simulink model "VTOL_V4_Final_LANDING"  (R2022b)
settings: Solver=ode23s  StartTime=0.0  StopTime=20  RelTol=1e-3
values from neighbouring files (symbols this model uses):
  x0 = [Cruise.landingConditions.uvw.Data(end,1) ... (first row only)    [Plot_Transition.m]    (also in Start.m = [21.9999986140590)
undefined symbols (not defined in the file or in its folder): F, Light, MIL
libraries: slpidlib x5, aerolibwind2 x2, shared6dof x1, aerolibatmos2 x1, simulink x1
settings Model: Creator=Jem  LastModifiedBy=Jem

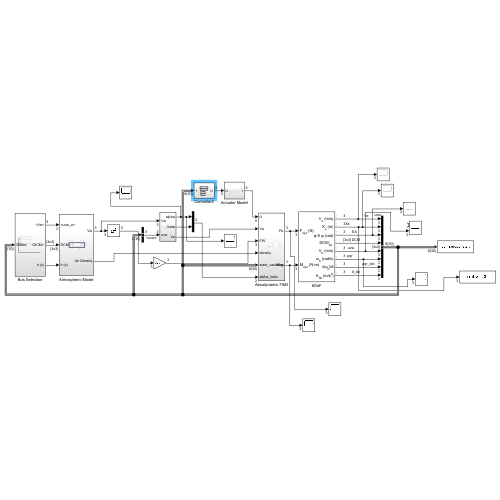
[thumbnail: Simulink's stored preview of the top-level diagram]
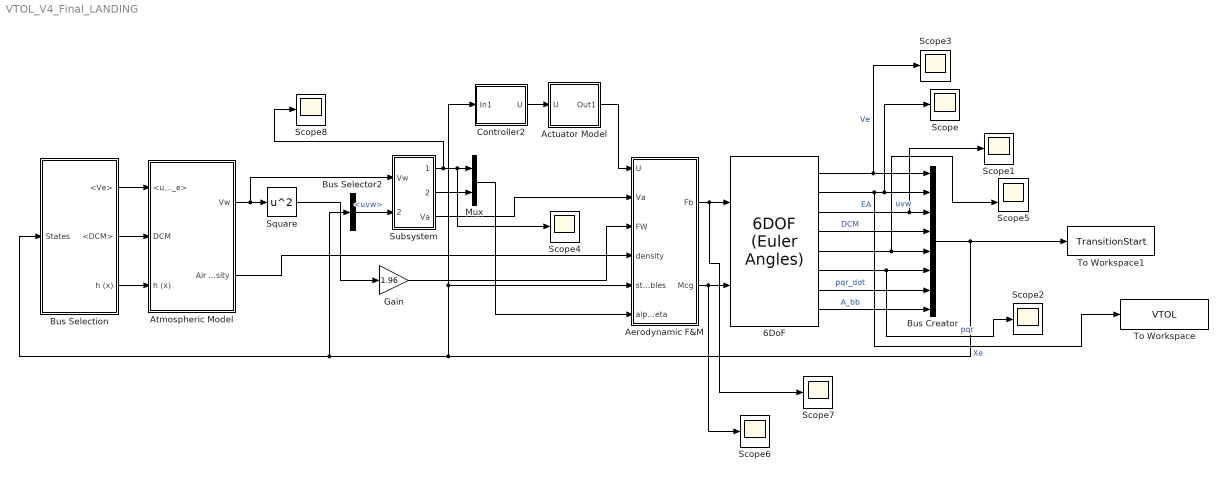
== system VTOL_V4_Final_LANDING ==
  6DoF : shared6dof/6DOF (Euler Angles)  units=Metric (MKS)  mtype=Fixed  rep=Euler Angles  xme_0=xyz0  Vm_0=x0(1:3)  eul_0=x0(7:9)  pm_0=x0(4:6)  mass_0=150  mass_e=0.5  mass_f=2.0  inertia=I  inertia_e=eye(3)  inertia_f=2*eye(3)  k_quat=1.0  vre_flag=on  abi_flag=off  aMode=0  xme_statename=''  Vm_statename=''  eul_statename=''  quat_statename=''  pm_statename=''  mass_statename=''
  Actuator Model : Subsystem
  Aerodynamic F&M : Subsystem
  Atmospheric Model : Subsystem
  Bus Creator : BusCreator  Inputs=8
  Bus Selector2 : BusSelector  OutputSignals=uvw
  Bus Selection : Subsystem
  Controller2 : Subsystem
  Gain : Gain  Gain=1.96
  Mux : Mux  Inputs=2
  Scope{,1..4,6..8} (8 alike) : Scope
  Scope5 : Scope  NumInputPorts=2
  Square : Math  Operator=square
  Subsystem : Subsystem
  To Workspace : ToWorkspace  VariableName=VTOL  SaveFormat=Timeseries  SampleTime=-1
  To Workspace1 : ToWorkspace  VariableName=TransitionStart  SaveFormat=Timeseries  SampleTime=-1
  wires:
  6DoF/3 -> Scope1/1, Bus Creator/3  "EA"
  6DoF/5 -> Scope5/2, Bus Creator/5  "uvw"
  6DoF/6 -> Scope2/1, Bus Creator/6  "pqr"
  6DoF/7 -> Bus Creator/7  "pqr_dot"
  6DoF/8 -> Bus Creator/8  "A_bb"
  6DoF/1 -> Scope3/1, Bus Creator/1  "Ve"
  Actuator Model/1(Out1) -> Aerodynamic F&M/1(U)
  Bus Creator/1 -> Aerodynamic F&M/5(state_variables), Controller2/1(In1), Bus Selection/1(States), Bus Selector2/1, To Workspace1/1
  6DoF/4 -> Bus Creator/4  "DCM"
  6DoF/2 -> To Workspace/1, Scope/1, Bus Creator/2  "Xe"
  Aerodynamic F&M/1(Fb) -> Scope7/1, 6DoF/1
  Bus Selector2/1 -> Subsystem/2(uvw)  "<uvw>"
  Bus Selection/1(<Ve>) -> Atmospheric Model/1(<uvw_e>)
  Atmospheric Model/2(Air Density) -> Aerodynamic F&M/4(density)
  Aerodynamic F&M/2(Mcg) -> Scope6/1, 6DoF/2
  Controller2/1(U) -> Actuator Model/1(U)
  Subsystem/3(Va) -> Aerodynamic F&M/2(Va)
  Subsystem/1(alpha) -> Scope8/1, Scope4/1, Mux/1
  Subsystem/2(beta) -> Mux/2
  Mux/1 -> Aerodynamic F&M/6(alpha_beta)
  Square/1 -> Gain/1
  Atmospheric Model/1(Vw) -> Subsystem/1(Vw), Square/1
  Bus Selection/3(h (x)) -> Atmospheric Model/3(h (x))
  Bus Selection/2(<DCM>) -> Atmospheric Model/2(DCM)
  Gain/1 -> Aerodynamic F&M/3(FW)

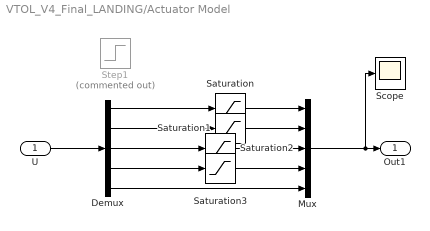
== system VTOL_V4_Final_LANDING/Actuator Model ==
  U : Inport
  Demux : Demux  Outputs=5
  Mux : Mux  Inputs=5
  Saturation{,1..3} (4 alike) : Saturate  UpperLimit=800  LowerLimit=0
  Scope : Scope
  Step1 : Step  Commented=on  Time=0.1  After=0.3629  SampleTime=0
  Out1 : Outport
  wires:
  Mux/1 -> Scope/1, Out1/1
  U/1 -> Demux/1
  Demux/1 -> Saturation/1
  Demux/2 -> Saturation1/1
  Demux/3 -> Saturation2/1
  Demux/4 -> Saturation3/1
  Demux/5 -> Mux/5
  Saturation/1 -> Mux/1
  Saturation1/1 -> Mux/2
  Saturation2/1 -> Mux/3
  Saturation3/1 -> Mux/4

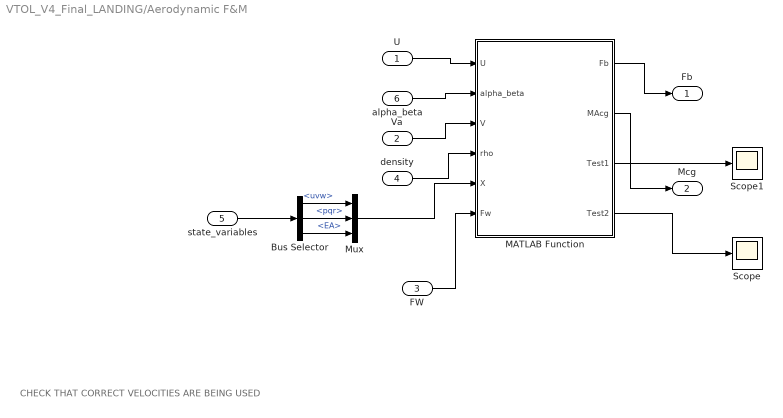
== system VTOL_V4_Final_LANDING/Aerodynamic F&M ==
  note: CHECK THAT CORRECT VELOCITIES ARE BEING USED
  U : Inport
  Va : Inport  Port=2
  FW : Inport  Port=3
  density : Inport  Port=4
  state_variables : Inport  Port=5
  alpha_beta : Inport  Port=6
  Bus Selector : BusSelector  OutputSignals=uvw,pqr,EA
  MATLAB Function : MATLAB Function  TreatAsAtomicUnit=on
  Mux : Mux  Inputs=3
  Scope : Scope
  Scope1 : Scope
  Fb : Outport
  Mcg : Outport  Port=2
  wires:
  U/1 -> MATLAB Function/1(U)
  Va/1 -> MATLAB Function/3(V)
  density/1 -> MATLAB Function/4(rho)
  Mux/1 -> MATLAB Function/5(X)
  state_variables/1 -> Bus Selector/1
  Bus Selector/3 -> Mux/3  "<EA>"
  MATLAB Function/1(Fb) -> Fb/1
  Bus Selector/1 -> Mux/1  "<uvw>"
  Bus Selector/2 -> Mux/2  "<pqr>"
  MATLAB Function/2(MAcg) -> Mcg/1
  FW/1 -> MATLAB Function/6(Fw)
  alpha_beta/1 -> MATLAB Function/2(alpha_beta)
  MATLAB Function/4(Test2) -> Scope/1
  MATLAB Function/3(Test1) -> Scope1/1

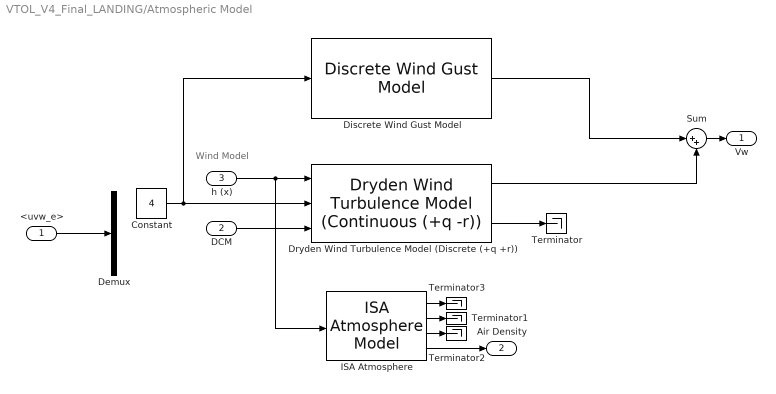
== system VTOL_V4_Final_LANDING/Atmospheric Model ==
  note: Wind Model
  <uvw_e> : Inport
  DCM : Inport  Port=2
  h (x) : Inport  Port=3
  Constant : Constant  Value=4
  Demux : Demux  Outputs=3
  Discrete Wind Gust Model : aerolibwind2/Discrete Wind Gust Model  units=Metric (MKS)  Gx=on  Gy=on  Gz=on  t_0=30  d_m=[120 120 80]  v_m=[6 6 6]
  Dryden Wind Turbulence Model (Discrete (+q +r)) : aerolibwind2/Dryden Wind Turbulence Model  (Continuous (+q -r))  units=Metric (MKS)  spec=MIL-F-8785C  model=Continuous Dryden (+q -r)  W20=6  Wdeg=8  TurbProb=10^-2 - Light  L_high=533.4  Wingspan=7  ts=0.1  Seed=[23341 23342 23343 23344]  T_on=on
      settings: LibrarySourceBlock=|
      | aerolibwind2/Dryden Wind Turbulence Model
      | (Discrete (+q +r))
  ISA Atmosphere : aerolibatmos2/ISA Atmosphere Model  custom=off  g=9.80665  gamma=1.4  R=287.0531  L=0.0065  h_trop=11000  h_strat=20000  rho0=1.225  P0=101325  T0=288.15  h0=0
  Sum : Sum  Inputs=|++
  Terminator{,1..3} (4 alike) : Terminator
  Vw : Outport
  Air Density : Outport  Port=2
  wires:
  ISA Atmosphere/1 -> Terminator3/1
  ISA Atmosphere/2 -> Terminator1/1
  ISA Atmosphere/3 -> Terminator2/1
  ISA Atmosphere/4 -> Air Density/1
  Dryden Wind Turbulence Model (Discrete (+q +r))/1 -> Sum/2
  Dryden Wind Turbulence Model (Discrete (+q +r))/2 -> Terminator/1
  <uvw_e>/1 -> Demux/1
  DCM/1 -> Dryden Wind Turbulence Model (Discrete (+q +r))/3
  h (x)/1 -> ISA Atmosphere/1, Dryden Wind Turbulence Model (Discrete (+q +r))/1
  Constant/1 -> Discrete Wind Gust Model/1, Dryden Wind Turbulence Model (Discrete (+q +r))/2
  Sum/1 -> Vw/1
  Discrete Wind Gust Model/1 -> Sum/1

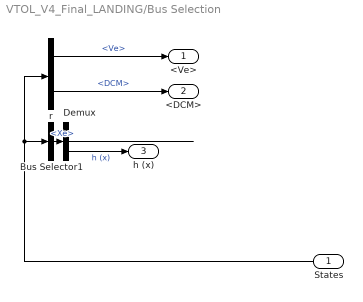
== system VTOL_V4_Final_LANDING/Bus Selection ==
  States : Inport
  Bus Selector1 : BusSelector  OutputSignals=Xe
  Demux : Demux  Outputs=3
  r : BusSelector  OutputSignals=Ve,DCM
  <Ve> : Outport
  <DCM> : Outport  Port=2
  h (x) : Outport  Port=3
  wires:
  r/1 -> <Ve>/1  "<Ve>"
  Demux/3 -> h (x)/1  "h (x)"
  Bus Selector1/1 -> Demux/1  "<Xe>"
  States/1 -> r/1, Bus Selector1/1
  r/2 -> <DCM>/1  "<DCM>"
  Demux/2 -> ?

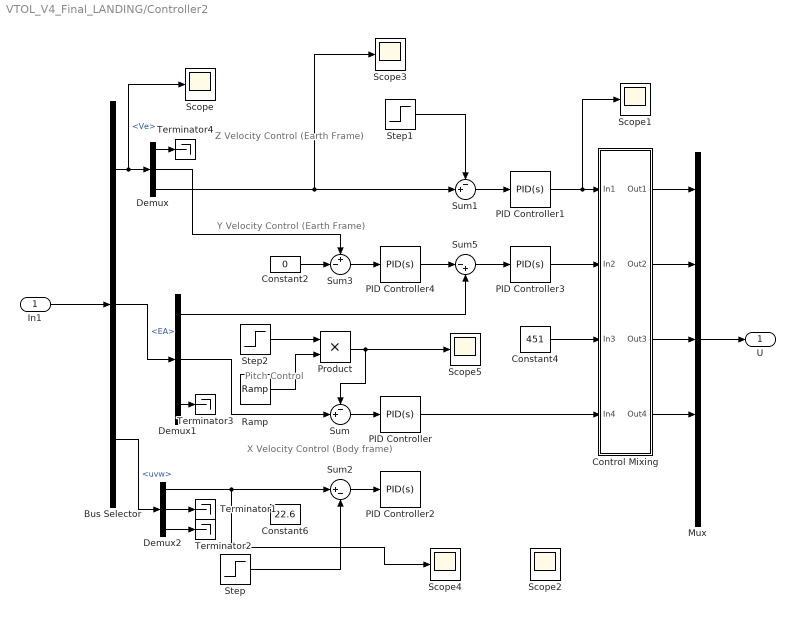
== system VTOL_V4_Final_LANDING/Controller2 ==
  note: Pitch Control
  note: X Velocity Control (Body frame)
  note: Y Velocity Control (Earth Frame)
  note: Z Velocity Control (Earth Frame)
  In1 : Inport
  Bus Selector : BusSelector  OutputSignals=Ve,EA,uvw
  Constant2 : Constant  Value=0
  Constant4 : Constant  Value=451
  Constant6 : Constant  Value=22.6
  Control Mixing : Subsystem
  Demux : Demux  Outputs=3
  Demux1 : Demux  Outputs=3
  Demux2 : Demux  Outputs=3
  Mux : Mux  Inputs=5
  PID Controller : slpidlib/PID Controller  Controller=PID  Form=Parallel  TimeDomain=Continuous-time  UseExternalTs=off  SampleTime=-1  IntegratorMethod=Forward Euler  FilterMethod=Forward Euler  ControllerParametersSource=internal  P=1329.62943172889  I=1105.82888130286  UseKiTs=off  D=392.472747796412  N=97.4795174075225  UseFilter=on  TunerSelectOption=Transfer Function Based (PID Tuner App)  InitialConditionSource=internal  InitialConditionForIntegrator=284.6  InitialConditionForFilter=200  DifferentiatorICPrevScaledInput=0  ExternalReset=none  TrackingMode=off  Kt=1  LimitOutput=on  SatLimitsSource=internal  UpperSaturationLimit=320  LowerSaturationLimit=200  LinearizeAsGain=on  AntiWindupMode=clamping  Kb=1  LimitIntegrator=off  UpperIntegratorSaturationLimit=inf  LowerIntegratorSaturationLimit=-inf  POutMin=[]  POutMax=[]  IOutMin=[]  IOutMax=[]  DOutMin=[]  DOutMax=[]  NOutMin=[]  NOutMax=[]  SumOutMin=[]  SumOutMax=[]  SaturationOutMin=[]  SaturationOutMax=[]  PParamMin=[]  PParamMax=[]  IParamMin=[]  IParamMax=[]  DParamMin=[]  DParamMax=[]  NParamMin=[]  NParamMax=[]  KbParamMin=[]  KbParamMax=[]  KtParamMin=[]  KtParamMax=[]  KbOutMin=[]  KbOutMax=[]  KtOutMin=[]  KtOutMax=[]  IntegratorOutMin=[]  IntegratorOutMax=[]  FilterOutMin=[]  FilterOutMax=[]  SumI1OutMin=[]  SumI1OutMax=[]  SumI2OutMin=[]  SumI2OutMax=[]  SumI3OutMin=[]  SumI3OutMax=[]  SumI4OutMin=[]  SumI4OutMax=[]  SumDOutMin=[]  SumDOutMax=[]  DifferentiatorOutMin=[]  DifferentiatorOutMax=[]  FilterDiffOutCoefMin=[]  FilterDiffOutCoefMax=[]  ReciprocalOutMin=[]  ReciprocalOutMax=[]  SumDenOutMin=[]  SumDenOutMax=[]  SumNumOutMin=[]  SumNumOutMax=[]  DivideOutMin=[]  DivideOutMax=[]  UdiffTsProdOutMin=[]  UdiffTsProdOutMax=[]  NTsProdOutMin=[]  NTsProdOutMax=[]  UintegralTsProdOutMin=[]  UintegralTsProdOutMax=[]  UngainTsProdOutMin=[]  UngainTsProdOutMax=[]  ClampingZeroOutDataTypeStr=Inherit: Inherit via back propagation  ClampingZeroOutMin=[]  ClampingZeroOutMax=[]  FilterDenConstantOutDataTypeStr=Inherit: Inherit via back propagation  FilterDenConstantOutMin=[]  FilterDenConstantOutMax=[]  PCopyOutDataTypeStr=Inherit: Inherit via back propagation  PCopyOutMin=[]  PCopyOutMax=[]  NCopyOutDataTypeStr=Inherit: Inherit via back propagation  NCopyOutMin=[]  NCopyOutMax=[]  IntegratorContinuousStateAttributes=''  IntegratorStateMustResolveToSignalObject=off  IntegratorRTWStateStorageClass=Auto  FilterContinuousStateAttributes=''  FilterStateMustResolveToSignalObject=off  FilterRTWStateStorageClass=Auto  ParallelPVariant=InternalParameters  IdealPVariant=Disabled  IVariant=InternalParameters  DVariant=InternalParameters  IntegratorVariant=Continuous  SatVariant=Enabled  AWVariant=ContClampingParallel  PCopyVariant=Disabled  TRVariant=Disabled  FdbkBlocksVariant=Forward  IdealPFdbkVariant=Disabled  SatFdbkVariant=Disabled  DerivativeFilterVariant=ContFilter  NVariant=InternalParameters  NCopyVariant=Disabled  FilterICVariant=InternalICsFilter  IntegratorICVariant=InternalICs  ExternalResetVariant=Disabled  TRSumVariant=Passthrough  SumFdbkVariant=Disabled  SumVariant=Sum_PID  TsampFilterVariant=InternalTs  TsampNgainVariant=Passthrough  TsampIntegralVariant=Passthrough  ExternalSaturationOutDataTypeStr=Inherit: Same as second input
  PID Controller1 : slpidlib/PID Controller  Controller=PID  Form=Parallel  TimeDomain=Continuous-time  UseExternalTs=off  SampleTime=-1  IntegratorMethod=Forward Euler  FilterMethod=Forward Euler  ControllerParametersSource=internal  P=4437.31089964675  I=78357.1615681682  UseKiTs=off  D=8.48105858167971  N=364.6824066771  UseFilter=on  TunerSelectOption=Transfer Function Based (PID Tuner App)  InitialConditionSource=internal  InitialConditionForIntegrator=25  InitialConditionForFilter=0  DifferentiatorICPrevScaledInput=0  ExternalReset=none  IgnoreLimit=on  TrackingMode=off  Kt=1  LimitOutput=on  SatLimitsSource=internal  UpperSaturationLimit=25  LowerSaturationLimit=-90  LinearizeAsGain=on  AntiWindupMode=clamping  Kb=1  LimitIntegrator=off  UpperIntegratorSaturationLimit=inf  LowerIntegratorSaturationLimit=-inf  POutMin=[]  POutMax=[]  IOutMin=[]  IOutMax=[]  DOutMin=[]  DOutMax=[]  NOutMin=[]  NOutMax=[]  SumOutMin=[]  SumOutMax=[]  SaturationOutMin=[]  SaturationOutMax=[]  PParamMin=[]  PParamMax=[]  IParamMin=[]  IParamMax=[]  DParamMin=[]  DParamMax=[]  NParamMin=[]  NParamMax=[]  KbParamMin=[]  KbParamMax=[]  KtParamMin=[]  KtParamMax=[]  KbOutMin=[]  KbOutMax=[]  KtOutMin=[]  KtOutMax=[]  IntegratorOutMin=[]  IntegratorOutMax=[]  FilterOutMin=[]  FilterOutMax=[]  SumI1OutMin=[]  SumI1OutMax=[]  SumI2OutMin=[]  SumI2OutMax=[]  SumI3OutMin=[]  SumI3OutMax=[]  SumI4OutMin=[]  SumI4OutMax=[]  SumDOutMin=[]  SumDOutMax=[]  DifferentiatorOutMin=[]  DifferentiatorOutMax=[]  FilterDiffOutCoefMin=[]  FilterDiffOutCoefMax=[]  ReciprocalOutMin=[]  ReciprocalOutMax=[]  SumDenOutMin=[]  SumDenOutMax=[]  SumNumOutMin=[]  SumNumOutMax=[]  DivideOutMin=[]  DivideOutMax=[]  UdiffTsProdOutMin=[]  UdiffTsProdOutMax=[]  NTsProdOutMin=[]  NTsProdOutMax=[]  UintegralTsProdOutMin=[]  UintegralTsProdOutMax=[]  UngainTsProdOutMin=[]  UngainTsProdOutMax=[]  ClampingZeroOutDataTypeStr=Inherit: Inherit via back propagation  ClampingZeroOutMin=[]  ClampingZeroOutMax=[]  FilterDenConstantOutDataTypeStr=Inherit: Inherit via back propagation  FilterDenConstantOutMin=[]  FilterDenConstantOutMax=[]  PCopyOutDataTypeStr=Inherit: Inherit via back propagation  PCopyOutMin=[]  PCopyOutMax=[]  NCopyOutDataTypeStr=Inherit: Inherit via back propagation  NCopyOutMin=[]  NCopyOutMax=[]  IntegratorContinuousStateAttributes=''  IntegratorStateMustResolveToSignalObject=off  IntegratorRTWStateStorageClass=Auto  FilterContinuousStateAttributes=''  FilterStateMustResolveToSignalObject=off  FilterRTWStateStorageClass=Auto  ParallelPVariant=InternalParameters  IdealPVariant=Disabled  IVariant=InternalParameters  DVariant=InternalParameters  IntegratorVariant=Continuous  SatVariant=Enabled  AWVariant=ContClampingParallel  PCopyVariant=Disabled  TRVariant=Disabled  FdbkBlocksVariant=Forward  IdealPFdbkVariant=Disabled  SatFdbkVariant=Disabled  DerivativeFilterVariant=ContFilter  NVariant=InternalParameters  NCopyVariant=Disabled  FilterICVariant=InternalICsFilter  IntegratorICVariant=InternalICs  ExternalResetVariant=Disabled  TRSumVariant=Passthrough  SumFdbkVariant=Disabled  SumVariant=Sum_PID  TsampFilterVariant=InternalTs  TsampNgainVariant=Passthrough  TsampIntegralVariant=Passthrough  ExternalSaturationOutDataTypeStr=Inherit: Same as second input
  PID Controller2 : slpidlib/PID Controller  Controller=PID  Form=Parallel  TimeDomain=Continuous-time  UseExternalTs=off  SampleTime=-1  IntegratorMethod=Forward Euler  FilterMethod=Forward Euler  ControllerParametersSource=internal  P=-640.079326699596  I=-549.524194779887  UseKiTs=off  D=54.1789709707112  N=11.8141654452171  UseFilter=on  TunerSelectOption=Transfer Function Based (PID Tuner App)  InitialConditionSource=internal  InitialConditionForIntegrator=0  InitialConditionForFilter=0  DifferentiatorICPrevScaledInput=0  ExternalReset=none  TrackingMode=off  Kt=1  LimitOutput=on  SatLimitsSource=internal  UpperSaturationLimit=300  LowerSaturationLimit=0  LinearizeAsGain=on  AntiWindupMode=clamping  Kb=1  LimitIntegrator=off  UpperIntegratorSaturationLimit=inf  LowerIntegratorSaturationLimit=-inf  POutMin=[]  POutMax=[]  IOutMin=[]  IOutMax=[]  DOutMin=[]  DOutMax=[]  NOutMin=[]  NOutMax=[]  SumOutMin=[]  SumOutMax=[]  SaturationOutMin=[]  SaturationOutMax=[]  PParamMin=[]  PParamMax=[]  IParamMin=[]  IParamMax=[]  DParamMin=[]  DParamMax=[]  NParamMin=[]  NParamMax=[]  KbParamMin=[]  KbParamMax=[]  KtParamMin=[]  KtParamMax=[]  KbOutMin=[]  KbOutMax=[]  KtOutMin=[]  KtOutMax=[]  IntegratorOutMin=[]  IntegratorOutMax=[]  FilterOutMin=[]  FilterOutMax=[]  SumI1OutMin=[]  SumI1OutMax=[]  SumI2OutMin=[]  SumI2OutMax=[]  SumI3OutMin=[]  SumI3OutMax=[]  SumI4OutMin=[]  SumI4OutMax=[]  SumDOutMin=[]  SumDOutMax=[]  DifferentiatorOutMin=[]  DifferentiatorOutMax=[]  FilterDiffOutCoefMin=[]  FilterDiffOutCoefMax=[]  ReciprocalOutMin=[]  ReciprocalOutMax=[]  SumDenOutMin=[]  SumDenOutMax=[]  SumNumOutMin=[]  SumNumOutMax=[]  DivideOutMin=[]  DivideOutMax=[]  UdiffTsProdOutMin=[]  UdiffTsProdOutMax=[]  NTsProdOutMin=[]  NTsProdOutMax=[]  UintegralTsProdOutMin=[]  UintegralTsProdOutMax=[]  UngainTsProdOutMin=[]  UngainTsProdOutMax=[]  ClampingZeroOutDataTypeStr=Inherit: Inherit via back propagation  ClampingZeroOutMin=[]  ClampingZeroOutMax=[]  FilterDenConstantOutDataTypeStr=Inherit: Inherit via back propagation  FilterDenConstantOutMin=[]  FilterDenConstantOutMax=[]  PCopyOutDataTypeStr=Inherit: Inherit via back propagation  PCopyOutMin=[]  PCopyOutMax=[]  NCopyOutDataTypeStr=Inherit: Inherit via back propagation  NCopyOutMin=[]  NCopyOutMax=[]  IntegratorContinuousStateAttributes=''  IntegratorStateMustResolveToSignalObject=off  IntegratorRTWStateStorageClass=Auto  FilterContinuousStateAttributes=''  FilterStateMustResolveToSignalObject=off  FilterRTWStateStorageClass=Auto  ParallelPVariant=InternalParameters  IdealPVariant=Disabled  IVariant=InternalParameters  DVariant=InternalParameters  IntegratorVariant=Continuous  SatVariant=Enabled  AWVariant=ContClampingParallel  PCopyVariant=Disabled  TRVariant=Disabled  FdbkBlocksVariant=Forward  IdealPFdbkVariant=Disabled  SatFdbkVariant=Disabled  DerivativeFilterVariant=ContFilter  NVariant=InternalParameters  NCopyVariant=Disabled  FilterICVariant=InternalICsFilter  IntegratorICVariant=InternalICs  ExternalResetVariant=Disabled  TRSumVariant=Passthrough  SumFdbkVariant=Disabled  SumVariant=Sum_PID  TsampFilterVariant=InternalTs  TsampNgainVariant=Passthrough  TsampIntegralVariant=Passthrough  ExternalSaturationOutDataTypeStr=Inherit: Same as second input
  PID Controller3 : slpidlib/PID Controller  Controller=PID  Form=Parallel  TimeDomain=Continuous-time  UseExternalTs=off  SampleTime=-1  IntegratorMethod=Forward Euler  FilterMethod=Forward Euler  ControllerParametersSource=internal  P=83.5732003293008  I=6.83324787919106  UseKiTs=off  D=247.166883076976  N=5.77982663752872  UseFilter=on  TunerSelectOption=Transfer Function Based (PID Tuner App)  InitialConditionSource=internal  InitialConditionForIntegrator=0  InitialConditionForFilter=0  DifferentiatorICPrevScaledInput=0  ExternalReset=none  TrackingMode=off  Kt=1  LimitOutput=on  SatLimitsSource=internal  UpperSaturationLimit=100  LowerSaturationLimit=-200  LinearizeAsGain=on  AntiWindupMode=clamping  Kb=1  LimitIntegrator=off  UpperIntegratorSaturationLimit=inf  LowerIntegratorSaturationLimit=-inf  POutMin=[]  POutMax=[]  IOutMin=[]  IOutMax=[]  DOutMin=[]  DOutMax=[]  NOutMin=[]  NOutMax=[]  SumOutMin=[]  SumOutMax=[]  SaturationOutMin=[]  SaturationOutMax=[]  PParamMin=[]  PParamMax=[]  IParamMin=[]  IParamMax=[]  DParamMin=[]  DParamMax=[]  NParamMin=[]  NParamMax=[]  KbParamMin=[]  KbParamMax=[]  KtParamMin=[]  KtParamMax=[]  KbOutMin=[]  KbOutMax=[]  KtOutMin=[]  KtOutMax=[]  IntegratorOutMin=[]  IntegratorOutMax=[]  FilterOutMin=[]  FilterOutMax=[]  SumI1OutMin=[]  SumI1OutMax=[]  SumI2OutMin=[]  SumI2OutMax=[]  SumI3OutMin=[]  SumI3OutMax=[]  SumI4OutMin=[]  SumI4OutMax=[]  SumDOutMin=[]  SumDOutMax=[]  DifferentiatorOutMin=[]  DifferentiatorOutMax=[]  FilterDiffOutCoefMin=[]  FilterDiffOutCoefMax=[]  ReciprocalOutMin=[]  ReciprocalOutMax=[]  SumDenOutMin=[]  SumDenOutMax=[]  SumNumOutMin=[]  SumNumOutMax=[]  DivideOutMin=[]  DivideOutMax=[]  UdiffTsProdOutMin=[]  UdiffTsProdOutMax=[]  NTsProdOutMin=[]  NTsProdOutMax=[]  UintegralTsProdOutMin=[]  UintegralTsProdOutMax=[]  UngainTsProdOutMin=[]  UngainTsProdOutMax=[]  ClampingZeroOutDataTypeStr=Inherit: Inherit via back propagation  ClampingZeroOutMin=[]  ClampingZeroOutMax=[]  FilterDenConstantOutDataTypeStr=Inherit: Inherit via back propagation  FilterDenConstantOutMin=[]  FilterDenConstantOutMax=[]  PCopyOutDataTypeStr=Inherit: Inherit via back propagation  PCopyOutMin=[]  PCopyOutMax=[]  NCopyOutDataTypeStr=Inherit: Inherit via back propagation  NCopyOutMin=[]  NCopyOutMax=[]  IntegratorContinuousStateAttributes=''  IntegratorStateMustResolveToSignalObject=off  IntegratorRTWStateStorageClass=Auto  FilterContinuousStateAttributes=''  FilterStateMustResolveToSignalObject=off  FilterRTWStateStorageClass=Auto  ParallelPVariant=InternalParameters  IdealPVariant=Disabled  IVariant=InternalParameters  DVariant=InternalParameters  IntegratorVariant=Continuous  SatVariant=Enabled  AWVariant=ContClampingParallel  PCopyVariant=Disabled  TRVariant=Disabled  FdbkBlocksVariant=Forward  IdealPFdbkVariant=Disabled  SatFdbkVariant=Disabled  DerivativeFilterVariant=ContFilter  NVariant=InternalParameters  NCopyVariant=Disabled  FilterICVariant=InternalICsFilter  IntegratorICVariant=InternalICs  ExternalResetVariant=Disabled  TRSumVariant=Passthrough  SumFdbkVariant=Disabled  SumVariant=Sum_PID  TsampFilterVariant=InternalTs  TsampNgainVariant=Passthrough  TsampIntegralVariant=Passthrough  ExternalSaturationOutDataTypeStr=Inherit: Same as second input
  PID Controller4 : slpidlib/PID Controller  Controller=PID  Form=Parallel  TimeDomain=Continuous-time  UseExternalTs=off  SampleTime=-1  IntegratorMethod=Forward Euler  FilterMethod=Forward Euler  ControllerParametersSource=internal  P=-0.225041080622864  I=-0.0643991652326462  UseKiTs=off  D=-0.154916049977412  N=326.418052833048  UseFilter=on  TunerSelectOption=Transfer Function Based (PID Tuner App)  InitialConditionSource=internal  InitialConditionForIntegrator=0  InitialConditionForFilter=0  DifferentiatorICPrevScaledInput=0  ExternalReset=none  TrackingMode=off  Kt=1  LimitOutput=on  SatLimitsSource=internal  UpperSaturationLimit=0.3  LowerSaturationLimit=-0.3  LinearizeAsGain=on  AntiWindupMode=none  Kb=1  LimitIntegrator=off  UpperIntegratorSaturationLimit=inf  LowerIntegratorSaturationLimit=-inf  POutMin=[]  POutMax=[]  IOutMin=[]  IOutMax=[]  DOutMin=[]  DOutMax=[]  NOutMin=[]  NOutMax=[]  SumOutMin=[]  SumOutMax=[]  SaturationOutMin=[]  SaturationOutMax=[]  PParamMin=[]  PParamMax=[]  IParamMin=[]  IParamMax=[]  DParamMin=[]  DParamMax=[]  NParamMin=[]  NParamMax=[]  KbParamMin=[]  KbParamMax=[]  KtParamMin=[]  KtParamMax=[]  KbOutMin=[]  KbOutMax=[]  KtOutMin=[]  KtOutMax=[]  IntegratorOutMin=[]  IntegratorOutMax=[]  FilterOutMin=[]  FilterOutMax=[]  SumI1OutMin=[]  SumI1OutMax=[]  SumI2OutMin=[]  SumI2OutMax=[]  SumI3OutMin=[]  SumI3OutMax=[]  SumI4OutMin=[]  SumI4OutMax=[]  SumDOutMin=[]  SumDOutMax=[]  DifferentiatorOutMin=[]  DifferentiatorOutMax=[]  FilterDiffOutCoefMin=[]  FilterDiffOutCoefMax=[]  ReciprocalOutMin=[]  ReciprocalOutMax=[]  SumDenOutMin=[]  SumDenOutMax=[]  SumNumOutMin=[]  SumNumOutMax=[]  DivideOutMin=[]  DivideOutMax=[]  UdiffTsProdOutMin=[]  UdiffTsProdOutMax=[]  NTsProdOutMin=[]  NTsProdOutMax=[]  UintegralTsProdOutMin=[]  UintegralTsProdOutMax=[]  UngainTsProdOutMin=[]  UngainTsProdOutMax=[]  ClampingZeroOutDataTypeStr=Inherit: Inherit via back propagation  ClampingZeroOutMin=[]  ClampingZeroOutMax=[]  FilterDenConstantOutDataTypeStr=Inherit: Inherit via back propagation  FilterDenConstantOutMin=[]  FilterDenConstantOutMax=[]  PCopyOutDataTypeStr=Inherit: Inherit via back propagation  PCopyOutMin=[]  PCopyOutMax=[]  NCopyOutDataTypeStr=Inherit: Inherit via back propagation  NCopyOutMin=[]  NCopyOutMax=[]  IntegratorContinuousStateAttributes=''  IntegratorStateMustResolveToSignalObject=off  IntegratorRTWStateStorageClass=Auto  FilterContinuousStateAttributes=''  FilterStateMustResolveToSignalObject=off  FilterRTWStateStorageClass=Auto  ParallelPVariant=InternalParameters  IdealPVariant=Disabled  IVariant=InternalParameters  DVariant=InternalParameters  IntegratorVariant=Continuous  SatVariant=Enabled  AWVariant=Passthrough  PCopyVariant=Disabled  TRVariant=Disabled  FdbkBlocksVariant=Forward  IdealPFdbkVariant=Disabled  SatFdbkVariant=Disabled  DerivativeFilterVariant=ContFilter  NVariant=InternalParameters  NCopyVariant=Disabled  FilterICVariant=InternalICsFilter  IntegratorICVariant=InternalICs  ExternalResetVariant=Disabled  TRSumVariant=Passthrough  SumFdbkVariant=Disabled  SumVariant=Sum_PID  TsampFilterVariant=InternalTs  TsampNgainVariant=Passthrough  TsampIntegralVariant=Passthrough  ExternalSaturationOutDataTypeStr=Inherit: Same as second input
  Product : Product
  Ramp : simulink/Sources/Ramp  slope=-0.1  start=13.5  InitialOutput=0.15
  Scope{,1..5} (6 alike) : Scope
  Step : Step  Time=0  After=0  SampleTime=0
  Step1 : Step  Time=8.05  Before=5.5  After=0  SampleTime=0
  Step2 : Step  Time=14.2  Before=1  After=0  SampleTime=0
  Sum : Sum  Inputs=-+|
  Sum1 : Sum  Inputs=-+|
  Sum2 : Sum  Inputs=|+-
  Sum3 : Sum  Inputs=+-|
  Sum5 : Sum  Inputs=|-+
  Terminator{1..4} (4 alike) : Terminator
  U : Outport
  wires:
  Sum/1 -> PID Controller/1
  In1/1 -> Bus Selector/1
  Bus Selector/1 -> Scope/1, Demux/1  "<Ve>"
  Bus Selector/2 -> Demux1/1  "<EA>"
  Mux/1 -> U/1
  Demux1/2 -> Sum/2
  Sum1/1 -> PID Controller1/1
  Sum2/1 -> PID Controller2/1
  Sum5/1 -> PID Controller3/1
  Control Mixing/1(Out1) -> Mux/1
  Control Mixing/2(Out2) -> Mux/2
  Control Mixing/3(Out3) -> Mux/3
  Control Mixing/4(Out4) -> Mux/4
  Bus Selector/3 -> Demux2/1  "<uvw>"
  Demux2/1 -> Scope4/1, Sum2/1
  Demux/3 -> Scope3/1, Sum1/2
  Demux1/1 -> Sum5/2
  PID Controller1/1 -> Scope1/1, Control Mixing/1(In1)
  Demux/2 -> Sum3/1
  Sum3/1 -> PID Controller4/1
  Constant4/1 -> Control Mixing/3(In3)
  PID Controller/1 -> Control Mixing/4(In4)
  PID Controller3/1 -> Control Mixing/2(In2)
  Demux2/2 -> Terminator1/1
  Demux2/3 -> Terminator2/1
  Demux1/3 -> Terminator3/1
  Demux/1 -> Terminator4/1
  Step1/1 -> Sum1/1
  PID Controller4/1 -> Sum5/1
  Constant2/1 -> Sum3/2
  Step/1 -> Sum2/2
  Step2/1 -> Product/1
  Product/1 -> Sum/1, Scope5/1
  Ramp/1 -> Product/2

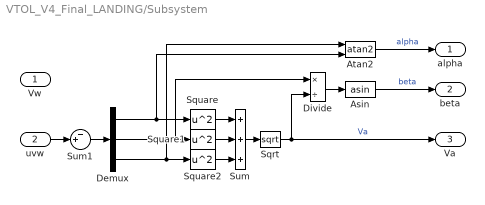
== system VTOL_V4_Final_LANDING/Subsystem ==
  Vw : Inport
  uvw : Inport  Port=2
  Asin : Trigonometry  Operator=asin
  Atan2 : Trigonometry  Operator=atan2
  Demux : Demux  Outputs=3
  Divide : Product  Inputs=*/
  Sqrt : Sqrt
  Square : Math  Operator=square
  Square1 : Math  Operator=square
  Square2 : Math  Operator=square
  Sum : Sum  Inputs=+++
  Sum1 : Sum  Inputs=-+|
  alpha : Outport
  beta : Outport  Port=2
  Va : Outport  Port=3
  wires:
  Square2/1 -> Sum/3
  Sum1/1 -> Demux/1
  Demux/2 -> Divide/1, Square1/1
  Demux/3 -> Square2/1, Atan2/1
  Square/1 -> Sum/1
  Square1/1 -> Sum/2
  Sqrt/1 -> Va/1, Divide/2  "Va"
  Divide/1 -> Asin/1
  Sum/1 -> Sqrt/1
  uvw/1 -> Sum1/2
  Atan2/1 -> alpha/1  "alpha"
  Asin/1 -> beta/1  "beta"
  Demux/1 -> Atan2/2, Square/1

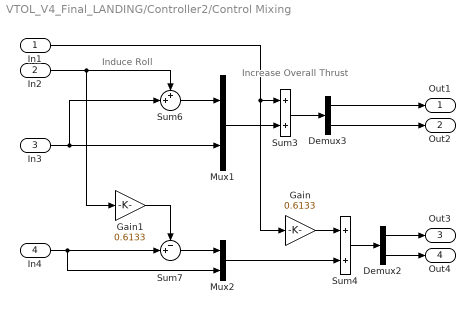
== system VTOL_V4_Final_LANDING/Controller2/Control Mixing ==
  note: Induce Roll
  note: Increase Overall Thrust
  In1 : Inport
  In2 : Inport  Port=2
  In3 : Inport  Port=3
  In4 : Inport  Port=4
  Demux2 : Demux  Outputs=2
  Demux3 : Demux  Outputs=2
  Gain : Gain  Gain=0.6133
  Gain1 : Gain  Gain=0.6133
  Mux1 : Mux  Inputs=2
  Mux2 : Mux  Inputs=2
  Sum3 : Sum
  Sum4 : Sum
  Sum6 : Sum  Inputs=++|
  Sum7 : Sum  Inputs=-+|
  Out1 : Outport
  Out2 : Outport  Port=2
  Out3 : Outport  Port=3
  Out4 : Outport  Port=4
  wires:
  Sum7/1 -> Mux2/1
  Sum4/1 -> Demux2/1
  In1/1 -> Gain/1, Sum3/1
  Sum6/1 -> Mux1/1
  In2/1 -> Sum6/1, Gain1/1
  Gain/1 -> Sum4/1
  Sum3/1 -> Demux3/1
  Mux1/1 -> Sum3/2
  In3/1 -> Sum6/2, Mux1/2
  Demux2/1 -> Out3/1
  Gain1/1 -> Sum7/1
  In4/1 -> Mux2/2, Sum7/2
  Mux2/1 -> Sum4/2
  Demux2/2 -> Out4/1
  Demux3/2 -> Out2/1
  Demux3/1 -> Out1/1

== matlab function VTOL_V4_Final_LANDING/Aerodynamic F&M/MATLAB Function ==
  data: U input; alpha_beta input; Fb output; V input; rho input; X input; MAcg output; Fw input; Test1 output; Test2 output
function [Fb, MAcg, Test1, Test2] = VTOL_6Dof(U, alpha_beta,V, rho, X, Fw)
% Function RCAM simulates ....
%
% Jemima Poynton 30/03/2023
% 
% Referenced against: https://www.youtube.com/watch?v=bFFAL9lI2IQ&t=3645s 
%% Setting up intermediate variables
% X(1:3) = X(1:3) - WB;
% V = sqrt(X(1)^2 + X(2)^2 + X(3)^2); % Total velocity
% alpha = atan2(X(3), X(1)); % AoA
% beta = asin(X(2)/V); % sideslip angle
% 
% rho = 1.167; % ASSUMPTION: ALTITUDE IS APPROXIMATELY CONSTANT IN CRUISE
alpha = alpha_beta(1);
beta = alpha_beta(2);
b = 7;

Q = 0.5*rho*V^2; % Dynamic pressure Q
a1 = 4.451;
a2 = 2.94;

Q = 0.5*rho*V^2; % Dynamic pressure Q
S = 8.34;
c = 1.46;
CM0 = -0.02;
m = 150;

%% Seperating vectors (BFR)
V_ = X(1:3); % Translational velocity vector
w_ = X(4:6); % Angular velocity vector

%% Vertical thrust from prop
T = U(1) + U(2) + U(3) + U(4);

%% Non-dimensional Aerodynamic Force Coefficients
% In stability axis frame Fs (RCAM Doc. Section 2.3.4)

% Wing-body nacelle lift
a = 3.72; % Lift-curve slope
n1 = -155.2; 
n2 = 609.2*n1;
n3 = -768.5;
n0 = 15.212; % Solve for n0 to solve discontinuity***
aL0 = -5*(pi/180);

if alpha <= 14.5*(pi/180) % ASSUMPTION: Cl is only a function of alpha
    Clwbn = a*(alpha - aL0);
else
    Clwbn = 0;
end

% Tail lift
lT = 1.95; %  [m] Tail moment arm NB: CG to AC (tail) NOT AC (wing) to AC (tail) %    [m]
S = 8.34; %    [m]
c = 1.46; %    [m]
m = 150; % [kg]
CM0 = -0.02;
etaT = 0.1009;
Vbar = 0.1320;
St = Vbar*S*c/lT;

dpr = 1.3*X(5)*lT/V; % Dynamic Pitch Response
epsilon = 0;
alphaT =  alpha - epsilon + dpr + etaT; % No downwash on canard

ClT = a1*alphaT; % Where does 3.1 come from??
CL = Clwbn + ClT;
if V < 15
    CL = 0
end

% Drag Model
CD = 0.018 + 0.062*(CL^2);

% Sideforce Coefficient
CY = -0.3381*beta; % Where will this empirical relationship come from?

%% Rotate from Fs to Fb (body axis)
TB = [U(5); 0; -T]; % Force vector in the stability frame

FAs = [-CD*S*Q; CY*Q*S; -CL*Q*S];

Cbs = [cos(alpha)*cos(beta), -cos(alpha)*sin(beta), -sin(alpha);  
       sin(beta)           ,  cos(beta)            ,  0         ; 
       cos(beta)*sin(alpha), -sin(alpha)*sin(beta),  cos(alpha)];

FAb = TB + Cbs*FAs;
%% Moment equations about CG
% in Fb

% Distances in each DoF
xfr_pitch = 1.2867;
xrr_pitch = 2.0383;

yrr_roll = 1.72;
yfr_roll = 1.72;

matT = [(U(2) - U(1))*yrr_roll - (U(3) - U(4))*yfr_roll;
        (U(1) + U(2))*xfr_pitch - (U(3) + U(4))*xrr_pitch;
        0];


%% Aerodynamic Moments
matA = [-0.1791*beta                      ;   % Equation of page 16 of the RCAM document, split into 3 terms
        CM0 + a1*Vbar*alphaT; 
        0.06724*beta]; 

Cmac = matA;

Mac = Cmac*Q*S.*[b;c;b];

r = [0.505;
     0     ;
     0     ]*c;

MAcg = Mac + cross(FAb, r); 

%% Gravity Effects
% Converted between earth frame and body frame

Fgb = [-9.81*sin(X(8))          ; % Body frame
        9.81*cos(X(8))*sin(X(7));
        9.81*cos(X(8))*cos(X(7))]*m; % ASSUMPTION: Constant Mass

% Moment about CG is zero

%% Explicit First Order Form
% Inertia matrix
Fb = Fgb + FAb;
MAcg = matT;
Test1 = FAb;
Test2 = TB;
